simulink model "Proiect"  (R2023b)
settings: Solver=ode45  StartTime=0.0  StopTime=3600  RelTol=1e-3
values from neighbouring files (symbols this model uses):
  A = 332.5    [Proiect.m]
  C = 5.75    [Proiect.m]
  h = 12.99    [Proiect.m]
  h0 = 10.22    [Proiect.m]
  k = 0.025    [Proiect.m]
  k1 = 0.654    [Proiect.m]
  k11 = k2^2 + 4 * (k - k3) * k1    (= 0.0671946)    [Proiect.m]
  k12 = 8 * (k - k3)    (= 0.2048)    [Proiect.m]
  k13 = 2 * (k - k3)    (= 0.0512)    [Proiect.m]
  k2 = -0.015    [Proiect.m]
  k3 = -0.0006    [Proiect.m]
  k_compensare = kpFF/kp_comp    (= 0.13698630137)    [Proiect.m]
  k_eta = 8 * 10^(-5)    (= 8e-05)    [Proiect.m]
  ki2 = 0.184    [Proiect.m]
  kr = 2.1661    [Proiect.m]
  kr1 = Tf1/(kf1*T01)    (= 0.30303030303)    [Proiect.m]
  kr2 = Tf2/(kf2*T02)    (= 47.4368231047)    [Proiect.m]
  kre2 = 47.4    [Proiect.m]
  kri2 = 0.303    [Proiect.m]
  q = 32.45    [Proiect.m]
  q0 = 28.8    [Proiect.m]
  Ti = kr * 1/0.01589    (= 136.31843927)    [Proiect.m]
  Tr1 = Tf1    (= 0.76)    [Proiect.m]
  Tr2 = Tf2    (= 258.25)    [Proiect.m]
  u0 = 4.5    [Proiect.m]
libraries: slpidlib x12
(part 1 of 2)
settings Model: Creator=raluc  LastModifiedBy=raluc
settings ModelReferenceCC: EnableRefExpFcnMdlSchedulingChecks=on

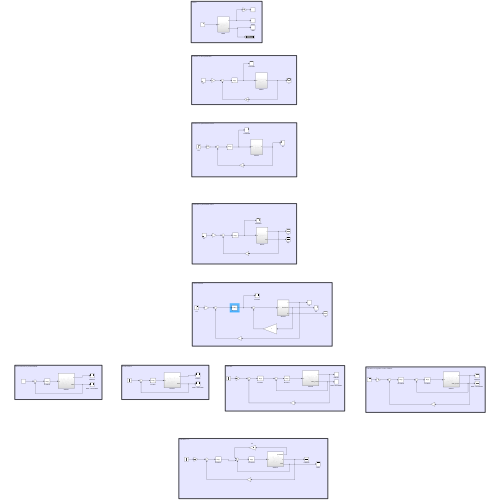
[thumbnail: Simulink's stored preview of the top-level diagram]
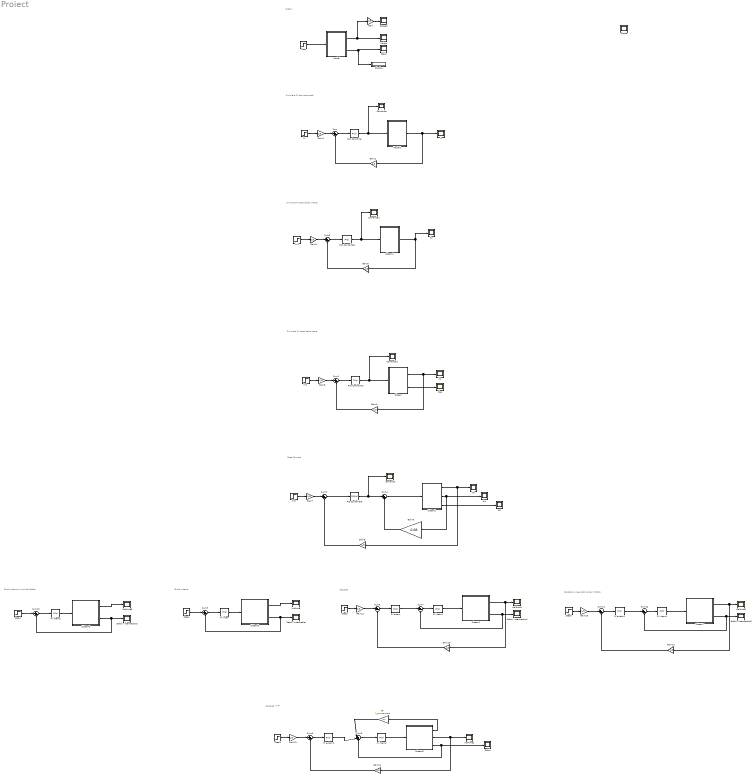
== system Proiect ==
  note: Cascada + FF
  note: Cascada
  note: Bucla Interna
  note: Feed Forward
  note: Simulare PI perturbatie intrare
  note: Simulare PI perturbatie iesire
  note: Simulare PI fara perturbatii
  note: Sistem
  note: Bucla Interna cu pid de Matlab
  note: Cascada cu regulator extern Matlab
  Comanda : Scope
  Comanda1 : Scope
  Comanda2 : Scope
  Debit : Scope
  Debit - intermediar{,1..3} (4 alike) : Scope
  Display : Display
  FF : Gain  Gain=k_compensare
  Gain{,1..8,10..15} (15 alike) : Gain  Gain=1/3
  Gain9 : Gain  Gain=0.08
  Inaltime{,1..4} (5 alike) : Scope
  Model : Subsystem
  Model1 : Subsystem
  PI extern : slpidlib/PID Controller  Controller=PI  Form=Parallel  TimeDomain=Continuous-time  UseExternalTs=off  SampleTime=-1  IntegratorMethod=Forward Euler  FilterMethod=Forward Euler  ControllerParametersSource=internal  P=kr2  I=kr2/Tr2  UseKiTs=off  D=0  N=100  UseFilter=on  TunerSelectOption=Transfer Function Based (PID Tuner App)  InitialConditionSource=internal  InitialConditionForIntegrator=q0  InitialConditionForFilter=0  DifferentiatorICPrevScaledInput=0  ExternalReset=none  TrackingMode=off  Kt=1  LimitOutput=off  SatLimitsSource=internal  UpperSaturationLimit=inf  LowerSaturationLimit=-inf  LinearizeAsGain=on  AntiWindupMode=none  Kb=1  LimitIntegrator=off  UpperIntegratorSaturationLimit=inf  LowerIntegratorSaturationLimit=-inf  POutMin=[]  POutMax=[]  IOutMin=[]  IOutMax=[]  DOutMin=[]  DOutMax=[]  NOutMin=[]  NOutMax=[]  SumOutMin=[]  SumOutMax=[]  SaturationOutMin=[]  SaturationOutMax=[]  PParamMin=[]  PParamMax=[]  IParamMin=[]  IParamMax=[]  DParamMin=[]  DParamMax=[]  NParamMin=[]  NParamMax=[]  KbParamMin=[]  KbParamMax=[]  KtParamMin=[]  KtParamMax=[]  KbOutMin=[]  KbOutMax=[]  KtOutMin=[]  KtOutMax=[]  IntegratorOutMin=[]  IntegratorOutMax=[]  FilterOutMin=[]  FilterOutMax=[]  SumI1OutMin=[]  SumI1OutMax=[]  SumI2OutMin=[]  SumI2OutMax=[]  SumI3OutMin=[]  SumI3OutMax=[]  SumI4OutMin=[]  SumI4OutMax=[]  SumDOutMin=[]  SumDOutMax=[]  DifferentiatorOutMin=[]  DifferentiatorOutMax=[]  FilterDiffOutCoefMin=[]  FilterDiffOutCoefMax=[]  ReciprocalOutMin=[]  ReciprocalOutMax=[]  SumDenOutMin=[]  SumDenOutMax=[]  SumNumOutMin=[]  SumNumOutMax=[]  DivideOutMin=[]  DivideOutMax=[]  UdiffTsProdOutMin=[]  UdiffTsProdOutMax=[]  NTsProdOutMin=[]  NTsProdOutMax=[]  UintegralTsProdOutMin=[]  UintegralTsProdOutMax=[]  UngainTsProdOutMin=[]  UngainTsProdOutMax=[]  ClampingZeroOutDataTypeStr=Inherit: Inherit via back propagation  ClampingZeroOutMin=[]  ClampingZeroOutMax=[]  FilterDenConstantOutDataTypeStr=Inherit: Inherit via back propagation  FilterDenConstantOutMin=[]  FilterDenConstantOutMax=[]  PCopyOutDataTypeStr=Inherit: Inherit via back propagation  PCopyOutMin=[]  PCopyOutMax=[]  NCopyOutDataTypeStr=Inherit: Inherit via back propagation  NCopyOutMin=[]  NCopyOutMax=[]  IntegratorContinuousStateAttributes=''  IntegratorStateMustResolveToSignalObject=off  IntegratorRTWStateStorageClass=Auto  FilterContinuousStateAttributes=''  FilterStateMustResolveToSignalObject=off  FilterRTWStateStorageClass=Auto  ParallelPVariant=InternalParameters  IdealPVariant=Disabled  IVariant=InternalParameters  DVariant=Disabled  IntegratorVariant=Continuous  SatVariant=Disabled  AWVariant=Passthrough  PCopyVariant=Disabled  TRVariant=Disabled  FdbkBlocksVariant=Forward  IdealPFdbkVariant=Disabled  SatFdbkVariant=Disabled  DerivativeFilterVariant=Disabled  NVariant=Disabled  NCopyVariant=Disabled_SignalSpec  FilterICVariant=Disabled  IntegratorICVariant=InternalICs  ExternalResetVariant=Disabled  TRSumVariant=Passthrough  SumFdbkVariant=Disabled  SumVariant=Sum_PI  TsampFilterVariant=InternalTs  TsampNgainVariant=Passthrough  TsampIntegralVariant=Disabled_SignalSpec  ExternalSaturationOutDataTypeStr=Inherit: Same as second input
  PI extern1 : slpidlib/PID Controller  Controller=PI  Form=Parallel  TimeDomain=Continuous-time  UseExternalTs=off  SampleTime=-1  IntegratorMethod=Forward Euler  FilterMethod=Forward Euler  ControllerParametersSource=internal  P=kre2  I=ki2  UseKiTs=off  D=0  N=100  UseFilter=on  TunerSelectOption=Transfer Function Based (PID Tuner App)  InitialConditionSource=internal  InitialConditionForIntegrator=q0  InitialConditionForFilter=0  DifferentiatorICPrevScaledInput=0  ExternalReset=none  TrackingMode=off  Kt=1  LimitOutput=off  SatLimitsSource=internal  UpperSaturationLimit=inf  LowerSaturationLimit=-inf  LinearizeAsGain=on  AntiWindupMode=none  Kb=1  LimitIntegrator=off  UpperIntegratorSaturationLimit=inf  LowerIntegratorSaturationLimit=-inf  POutMin=[]  POutMax=[]  IOutMin=[]  IOutMax=[]  DOutMin=[]  DOutMax=[]  NOutMin=[]  NOutMax=[]  SumOutMin=[]  SumOutMax=[]  SaturationOutMin=[]  SaturationOutMax=[]  PParamMin=[]  PParamMax=[]  IParamMin=[]  IParamMax=[]  DParamMin=[]  DParamMax=[]  NParamMin=[]  NParamMax=[]  KbParamMin=[]  KbParamMax=[]  KtParamMin=[]  KtParamMax=[]  KbOutMin=[]  KbOutMax=[]  KtOutMin=[]  KtOutMax=[]  IntegratorOutMin=[]  IntegratorOutMax=[]  FilterOutMin=[]  FilterOutMax=[]  SumI1OutMin=[]  SumI1OutMax=[]  SumI2OutMin=[]  SumI2OutMax=[]  SumI3OutMin=[]  SumI3OutMax=[]  SumI4OutMin=[]  SumI4OutMax=[]  SumDOutMin=[]  SumDOutMax=[]  DifferentiatorOutMin=[]  DifferentiatorOutMax=[]  FilterDiffOutCoefMin=[]  FilterDiffOutCoefMax=[]  ReciprocalOutMin=[]  ReciprocalOutMax=[]  SumDenOutMin=[]  SumDenOutMax=[]  SumNumOutMin=[]  SumNumOutMax=[]  DivideOutMin=[]  DivideOutMax=[]  UdiffTsProdOutMin=[]  UdiffTsProdOutMax=[]  NTsProdOutMin=[]  NTsProdOutMax=[]  UintegralTsProdOutMin=[]  UintegralTsProdOutMax=[]  UngainTsProdOutMin=[]  UngainTsProdOutMax=[]  ClampingZeroOutDataTypeStr=Inherit: Inherit via back propagation  ClampingZeroOutMin=[]  ClampingZeroOutMax=[]  FilterDenConstantOutDataTypeStr=Inherit: Inherit via back propagation  FilterDenConstantOutMin=[]  FilterDenConstantOutMax=[]  PCopyOutDataTypeStr=Inherit: Inherit via back propagation  PCopyOutMin=[]  PCopyOutMax=[]  NCopyOutDataTypeStr=Inherit: Inherit via back propagation  NCopyOutMin=[]  NCopyOutMax=[]  IntegratorContinuousStateAttributes=''  IntegratorStateMustResolveToSignalObject=off  IntegratorRTWStateStorageClass=Auto  FilterContinuousStateAttributes=''  FilterStateMustResolveToSignalObject=off  FilterRTWStateStorageClass=Auto  ParallelPVariant=InternalParameters  IdealPVariant=Disabled  IVariant=InternalParameters  DVariant=Disabled  IntegratorVariant=Continuous  SatVariant=Disabled  AWVariant=Passthrough  PCopyVariant=Disabled  TRVariant=Disabled  FdbkBlocksVariant=Forward  IdealPFdbkVariant=Disabled  SatFdbkVariant=Disabled  DerivativeFilterVariant=Disabled  NVariant=Disabled  NCopyVariant=Disabled_SignalSpec  FilterICVariant=Disabled  IntegratorICVariant=InternalICs  ExternalResetVariant=Disabled  TRSumVariant=Passthrough  SumFdbkVariant=Disabled  SumVariant=Sum_PI  TsampFilterVariant=InternalTs  TsampNgainVariant=Passthrough  TsampIntegralVariant=Disabled_SignalSpec  ExternalSaturationOutDataTypeStr=Inherit: Same as second input
  PI extern2 : slpidlib/PID Controller  Controller=PI  Form=Parallel  TimeDomain=Continuous-time  UseExternalTs=off  SampleTime=-1  IntegratorMethod=Forward Euler  FilterMethod=Forward Euler  ControllerParametersSource=internal  P=kre2  I=ki2  UseKiTs=off  D=0  N=100  UseFilter=on  TunerSelectOption=Transfer Function Based (PID Tuner App)  InitialConditionSource=internal  InitialConditionForIntegrator=q0  InitialConditionForFilter=0  DifferentiatorICPrevScaledInput=0  ExternalReset=none  TrackingMode=off  Kt=1  LimitOutput=off  SatLimitsSource=internal  UpperSaturationLimit=inf  LowerSaturationLimit=-inf  LinearizeAsGain=on  AntiWindupMode=none  Kb=1  LimitIntegrator=off  UpperIntegratorSaturationLimit=inf  LowerIntegratorSaturationLimit=-inf  POutMin=[]  POutMax=[]  IOutMin=[]  IOutMax=[]  DOutMin=[]  DOutMax=[]  NOutMin=[]  NOutMax=[]  SumOutMin=[]  SumOutMax=[]  SaturationOutMin=[]  SaturationOutMax=[]  PParamMin=[]  PParamMax=[]  IParamMin=[]  IParamMax=[]  DParamMin=[]  DParamMax=[]  NParamMin=[]  NParamMax=[]  KbParamMin=[]  KbParamMax=[]  KtParamMin=[]  KtParamMax=[]  KbOutMin=[]  KbOutMax=[]  KtOutMin=[]  KtOutMax=[]  IntegratorOutMin=[]  IntegratorOutMax=[]  FilterOutMin=[]  FilterOutMax=[]  SumI1OutMin=[]  SumI1OutMax=[]  SumI2OutMin=[]  SumI2OutMax=[]  SumI3OutMin=[]  SumI3OutMax=[]  SumI4OutMin=[]  SumI4OutMax=[]  SumDOutMin=[]  SumDOutMax=[]  DifferentiatorOutMin=[]  DifferentiatorOutMax=[]  FilterDiffOutCoefMin=[]  FilterDiffOutCoefMax=[]  ReciprocalOutMin=[]  ReciprocalOutMax=[]  SumDenOutMin=[]  SumDenOutMax=[]  SumNumOutMin=[]  SumNumOutMax=[]  DivideOutMin=[]  DivideOutMax=[]  UdiffTsProdOutMin=[]  UdiffTsProdOutMax=[]  NTsProdOutMin=[]  NTsProdOutMax=[]  UintegralTsProdOutMin=[]  UintegralTsProdOutMax=[]  UngainTsProdOutMin=[]  UngainTsProdOutMax=[]  ClampingZeroOutDataTypeStr=Inherit: Inherit via back propagation  ClampingZeroOutMin=[]  ClampingZeroOutMax=[]  FilterDenConstantOutDataTypeStr=Inherit: Inherit via back propagation  FilterDenConstantOutMin=[]  FilterDenConstantOutMax=[]  PCopyOutDataTypeStr=Inherit: Inherit via back propagation  PCopyOutMin=[]  PCopyOutMax=[]  NCopyOutDataTypeStr=Inherit: Inherit via back propagation  NCopyOutMin=[]  NCopyOutMax=[]  IntegratorContinuousStateAttributes=''  IntegratorStateMustResolveToSignalObject=off  IntegratorRTWStateStorageClass=Auto  FilterContinuousStateAttributes=''  FilterStateMustResolveToSignalObject=off  FilterRTWStateStorageClass=Auto  ParallelPVariant=InternalParameters  IdealPVariant=Disabled  IVariant=InternalParameters  DVariant=Disabled  IntegratorVariant=Continuous  SatVariant=Disabled  AWVariant=Passthrough  PCopyVariant=Disabled  TRVariant=Disabled  FdbkBlocksVariant=Forward  IdealPFdbkVariant=Disabled  SatFdbkVariant=Disabled  DerivativeFilterVariant=Disabled  NVariant=Disabled  NCopyVariant=Disabled_SignalSpec  FilterICVariant=Disabled  IntegratorICVariant=InternalICs  ExternalResetVariant=Disabled  TRSumVariant=Passthrough  SumFdbkVariant=Disabled  SumVariant=Sum_PI  TsampFilterVariant=InternalTs  TsampNgainVariant=Passthrough  TsampIntegralVariant=Disabled_SignalSpec  ExternalSaturationOutDataTypeStr=Inherit: Same as second input
  PI intern{,1..2,4} (4 alike) : slpidlib/PID Controller  Controller=PI  Form=Parallel  TimeDomain=Continuous-time  UseExternalTs=off  SampleTime=-1  IntegratorMethod=Forward Euler  FilterMethod=Forward Euler  ControllerParametersSource=internal  P=kr1  I=kr1/Tr1  UseKiTs=off  D=0  N=100  UseFilter=on  TunerSelectOption=Transfer Function Based (PID Tuner App)  InitialConditionSource=internal  InitialConditionForIntegrator=4.5  InitialConditionForFilter=0  DifferentiatorICPrevScaledInput=0  ExternalReset=none  TrackingMode=off  Kt=1  LimitOutput=off  SatLimitsSource=internal  UpperSaturationLimit=inf  LowerSaturationLimit=-inf  LinearizeAsGain=on  AntiWindupMode=none  Kb=1  LimitIntegrator=off  UpperIntegratorSaturationLimit=inf  LowerIntegratorSaturationLimit=-inf  POutMin=[]  POutMax=[]  IOutMin=[]  IOutMax=[]  DOutMin=[]  DOutMax=[]  NOutMin=[]  NOutMax=[]  SumOutMin=[]  SumOutMax=[]  SaturationOutMin=[]  SaturationOutMax=[]  PParamMin=[]  PParamMax=[]  IParamMin=[]  IParamMax=[]  DParamMin=[]  DParamMax=[]  NParamMin=[]  NParamMax=[]  KbParamMin=[]  KbParamMax=[]  KtParamMin=[]  KtParamMax=[]  KbOutMin=[]  KbOutMax=[]  KtOutMin=[]  KtOutMax=[]  IntegratorOutMin=[]  IntegratorOutMax=[]  FilterOutMin=[]  FilterOutMax=[]  SumI1OutMin=[]  SumI1OutMax=[]  SumI2OutMin=[]  SumI2OutMax=[]  SumI3OutMin=[]  SumI3OutMax=[]  SumI4OutMin=[]  SumI4OutMax=[]  SumDOutMin=[]  SumDOutMax=[]  DifferentiatorOutMin=[]  DifferentiatorOutMax=[]  FilterDiffOutCoefMin=[]  FilterDiffOutCoefMax=[]  ReciprocalOutMin=[]  ReciprocalOutMax=[]  SumDenOutMin=[]  SumDenOutMax=[]  SumNumOutMin=[]  SumNumOutMax=[]  DivideOutMin=[]  DivideOutMax=[]  UdiffTsProdOutMin=[]  UdiffTsProdOutMax=[]  NTsProdOutMin=[]  NTsProdOutMax=[]  UintegralTsProdOutMin=[]  UintegralTsProdOutMax=[]  UngainTsProdOutMin=[]  UngainTsProdOutMax=[]  ClampingZeroOutDataTypeStr=Inherit: Inherit via back propagation  ClampingZeroOutMin=[]  ClampingZeroOutMax=[]  FilterDenConstantOutDataTypeStr=Inherit: Inherit via back propagation  FilterDenConstantOutMin=[]  FilterDenConstantOutMax=[]  PCopyOutDataTypeStr=Inherit: Inherit via back propagation  PCopyOutMin=[]  PCopyOutMax=[]  NCopyOutDataTypeStr=Inherit: Inherit via back propagation  NCopyOutMin=[]  NCopyOutMax=[]  IntegratorContinuousStateAttributes=''  IntegratorStateMustResolveToSignalObject=off  IntegratorRTWStateStorageClass=Auto  FilterContinuousStateAttributes=''  FilterStateMustResolveToSignalObject=off  FilterRTWStateStorageClass=Auto  ParallelPVariant=InternalParameters  IdealPVariant=Disabled  IVariant=InternalParameters  DVariant=Disabled  IntegratorVariant=Continuous  SatVariant=Disabled  AWVariant=Passthrough  PCopyVariant=Disabled  TRVariant=Disabled  FdbkBlocksVariant=Forward  IdealPFdbkVariant=Disabled  SatFdbkVariant=Disabled  DerivativeFilterVariant=Disabled  NVariant=Disabled  NCopyVariant=Disabled_SignalSpec  FilterICVariant=Disabled  IntegratorICVariant=InternalICs  ExternalResetVariant=Disabled  TRSumVariant=Passthrough  SumFdbkVariant=Disabled  SumVariant=Sum_PI  TsampFilterVariant=InternalTs  TsampNgainVariant=Passthrough  TsampIntegralVariant=Disabled_SignalSpec  ExternalSaturationOutDataTypeStr=Inherit: Same as second input
  PI intern3 : slpidlib/PID Controller  Controller=PI  Form=Parallel  TimeDomain=Continuous-time  UseExternalTs=off  SampleTime=-1  IntegratorMethod=Forward Euler  FilterMethod=Forward Euler  ControllerParametersSource=internal  P=kri2  I=ki2  UseKiTs=off  D=0  N=100  UseFilter=on  TunerSelectOption=Transfer Function Based (PID Tuner App)  InitialConditionSource=internal  InitialConditionForIntegrator=4.5  InitialConditionForFilter=0  DifferentiatorICPrevScaledInput=0  ExternalReset=none  TrackingMode=off  Kt=1  LimitOutput=off  SatLimitsSource=internal  UpperSaturationLimit=inf  LowerSaturationLimit=-inf  LinearizeAsGain=on  AntiWindupMode=none  Kb=1  LimitIntegrator=off  UpperIntegratorSaturationLimit=inf  LowerIntegratorSaturationLimit=-inf  POutMin=[]  POutMax=[]  IOutMin=[]  IOutMax=[]  DOutMin=[]  DOutMax=[]  NOutMin=[]  NOutMax=[]  SumOutMin=[]  SumOutMax=[]  SaturationOutMin=[]  SaturationOutMax=[]  PParamMin=[]  PParamMax=[]  IParamMin=[]  IParamMax=[]  DParamMin=[]  DParamMax=[]  NParamMin=[]  NParamMax=[]  KbParamMin=[]  KbParamMax=[]  KtParamMin=[]  KtParamMax=[]  KbOutMin=[]  KbOutMax=[]  KtOutMin=[]  KtOutMax=[]  IntegratorOutMin=[]  IntegratorOutMax=[]  FilterOutMin=[]  FilterOutMax=[]  SumI1OutMin=[]  SumI1OutMax=[]  SumI2OutMin=[]  SumI2OutMax=[]  SumI3OutMin=[]  SumI3OutMax=[]  SumI4OutMin=[]  SumI4OutMax=[]  SumDOutMin=[]  SumDOutMax=[]  DifferentiatorOutMin=[]  DifferentiatorOutMax=[]  FilterDiffOutCoefMin=[]  FilterDiffOutCoefMax=[]  ReciprocalOutMin=[]  ReciprocalOutMax=[]  SumDenOutMin=[]  SumDenOutMax=[]  SumNumOutMin=[]  SumNumOutMax=[]  DivideOutMin=[]  DivideOutMax=[]  UdiffTsProdOutMin=[]  UdiffTsProdOutMax=[]  NTsProdOutMin=[]  NTsProdOutMax=[]  UintegralTsProdOutMin=[]  UintegralTsProdOutMax=[]  UngainTsProdOutMin=[]  UngainTsProdOutMax=[]  ClampingZeroOutDataTypeStr=Inherit: Inherit via back propagation  ClampingZeroOutMin=[]  ClampingZeroOutMax=[]  FilterDenConstantOutDataTypeStr=Inherit: Inherit via back propagation  FilterDenConstantOutMin=[]  FilterDenConstantOutMax=[]  PCopyOutDataTypeStr=Inherit: Inherit via back propagation  PCopyOutMin=[]  PCopyOutMax=[]  NCopyOutDataTypeStr=Inherit: Inherit via back propagation  NCopyOutMin=[]  NCopyOutMax=[]  IntegratorContinuousStateAttributes=''  IntegratorStateMustResolveToSignalObject=off  IntegratorRTWStateStorageClass=Auto  FilterContinuousStateAttributes=''  FilterStateMustResolveToSignalObject=off  FilterRTWStateStorageClass=Auto  ParallelPVariant=InternalParameters  IdealPVariant=Disabled  IVariant=InternalParameters  DVariant=Disabled  IntegratorVariant=Continuous  SatVariant=Disabled  AWVariant=Passthrough  PCopyVariant=Disabled  TRVariant=Disabled  FdbkBlocksVariant=Forward  IdealPFdbkVariant=Disabled  SatFdbkVariant=Disabled  DerivativeFilterVariant=Disabled  NVariant=Disabled  NCopyVariant=Disabled_SignalSpec  FilterICVariant=Disabled  IntegratorICVariant=InternalICs  ExternalResetVariant=Disabled  TRSumVariant=Passthrough  SumFdbkVariant=Disabled  SumVariant=Sum_PI  TsampFilterVariant=InternalTs  TsampNgainVariant=Passthrough  TsampIntegralVariant=Disabled_SignalSpec  ExternalSaturationOutDataTypeStr=Inherit: Same as second input
  PID Controller : slpidlib/PID Controller  Controller=PI  Form=Parallel  TimeDomain=Continuous-time  UseExternalTs=off  SampleTime=-1  IntegratorMethod=Forward Euler  FilterMethod=Forward Euler  ControllerParametersSource=internal  P=kr  I=kr/Ti  UseKiTs=off  D=0  N=100  UseFilter=on  TunerSelectOption=Transfer Function Based (PID Tuner App)  InitialConditionSource=internal  InitialConditionForIntegrator=u0  InitialConditionForFilter=0  DifferentiatorICPrevScaledInput=0  ExternalReset=none  TrackingMode=off  Kt=1  LimitOutput=off  SatLimitsSource=internal  UpperSaturationLimit=inf  LowerSaturationLimit=-inf  LinearizeAsGain=on  AntiWindupMode=none  Kb=1  LimitIntegrator=off  UpperIntegratorSaturationLimit=inf  LowerIntegratorSaturationLimit=-inf  POutMin=[]  POutMax=[]  IOutMin=[]  IOutMax=[]  DOutMin=[]  DOutMax=[]  NOutMin=[]  NOutMax=[]  SumOutMin=[]  SumOutMax=[]  SaturationOutMin=[]  SaturationOutMax=[]  PParamMin=[]  PParamMax=[]  IParamMin=[]  IParamMax=[]  DParamMin=[]  DParamMax=[]  NParamMin=[]  NParamMax=[]  KbParamMin=[]  KbParamMax=[]  KtParamMin=[]  KtParamMax=[]  KbOutMin=[]  KbOutMax=[]  KtOutMin=[]  KtOutMax=[]  IntegratorOutMin=[]  IntegratorOutMax=[]  FilterOutMin=[]  FilterOutMax=[]  SumI1OutMin=[]  SumI1OutMax=[]  SumI2OutMin=[]  SumI2OutMax=[]  SumI3OutMin=[]  SumI3OutMax=[]  SumI4OutMin=[]  SumI4OutMax=[]  SumDOutMin=[]  SumDOutMax=[]  DifferentiatorOutMin=[]  DifferentiatorOutMax=[]  FilterDiffOutCoefMin=[]  FilterDiffOutCoefMax=[]  ReciprocalOutMin=[]  ReciprocalOutMax=[]  SumDenOutMin=[]  SumDenOutMax=[]  SumNumOutMin=[]  SumNumOutMax=[]  DivideOutMin=[]  DivideOutMax=[]  UdiffTsProdOutMin=[]  UdiffTsProdOutMax=[]  NTsProdOutMin=[]  NTsProdOutMax=[]  UintegralTsProdOutMin=[]  UintegralTsProdOutMax=[]  UngainTsProdOutMin=[]  UngainTsProdOutMax=[]  ClampingZeroOutDataTypeStr=Inherit: Inherit via back propagation  ClampingZeroOutMin=[]  ClampingZeroOutMax=[]  FilterDenConstantOutDataTypeStr=Inherit: Inherit via back propagation  FilterDenConstantOutMin=[]  FilterDenConstantOutMax=[]  PCopyOutDataTypeStr=Inherit: Inherit via back propagation  PCopyOutMin=[]  PCopyOutMax=[]  NCopyOutDataTypeStr=Inherit: Inherit via back propagation  NCopyOutMin=[]  NCopyOutMax=[]  IntegratorContinuousStateAttributes=''  IntegratorStateMustResolveToSignalObject=off  IntegratorRTWStateStorageClass=Auto  FilterContinuousStateAttributes=''  FilterStateMustResolveToSignalObject=off  FilterRTWStateStorageClass=Auto  ParallelPVariant=InternalParameters  IdealPVariant=Disabled  IVariant=InternalParameters  DVariant=Disabled  IntegratorVariant=Continuous  SatVariant=Disabled  AWVariant=Passthrough  PCopyVariant=Disabled  TRVariant=Disabled  FdbkBlocksVariant=Forward  IdealPFdbkVariant=Disabled  SatFdbkVariant=Disabled  DerivativeFilterVariant=Disabled  NVariant=Disabled  NCopyVariant=Disabled_SignalSpec  FilterICVariant=Disabled  IntegratorICVariant=InternalICs  ExternalResetVariant=Disabled  TRSumVariant=Passthrough  SumFdbkVariant=Disabled  SumVariant=Sum_PI  TsampFilterVariant=InternalTs  TsampNgainVariant=Passthrough  TsampIntegralVariant=Disabled_SignalSpec  ExternalSaturationOutDataTypeStr=Inherit: Same as second input
  PID Controller1 : slpidlib/PID Controller  Controller=PI  Form=Parallel  TimeDomain=Continuous-time  UseExternalTs=off  SampleTime=-1  IntegratorMethod=Forward Euler  FilterMethod=Forward Euler  ControllerParametersSource=internal  P=kr  I=kr/Ti  UseKiTs=off  D=0  N=100  UseFilter=on  TunerSelectOption=Transfer Function Based (PID Tuner App)  InitialConditionSource=internal  InitialConditionForIntegrator=4.5  InitialConditionForFilter=0  DifferentiatorICPrevScaledInput=0  ExternalReset=none  TrackingMode=off  Kt=1  LimitOutput=off  SatLimitsSource=internal  UpperSaturationLimit=inf  LowerSaturationLimit=-inf  LinearizeAsGain=on  AntiWindupMode=none  Kb=1  LimitIntegrator=off  UpperIntegratorSaturationLimit=inf  LowerIntegratorSaturationLimit=-inf  POutMin=[]  POutMax=[]  IOutMin=[]  IOutMax=[]  DOutMin=[]  DOutMax=[]  NOutMin=[]  NOutMax=[]  SumOutMin=[]  SumOutMax=[]  SaturationOutMin=[]  SaturationOutMax=[]  PParamMin=[]  PParamMax=[]  IParamMin=[]  IParamMax=[]  DParamMin=[]  DParamMax=[]  NParamMin=[]  NParamMax=[]  KbParamMin=[]  KbParamMax=[]  KtParamMin=[]  KtParamMax=[]  KbOutMin=[]  KbOutMax=[]  KtOutMin=[]  KtOutMax=[]  IntegratorOutMin=[]  IntegratorOutMax=[]  FilterOutMin=[]  FilterOutMax=[]  SumI1OutMin=[]  SumI1OutMax=[]  SumI2OutMin=[]  SumI2OutMax=[]  SumI3OutMin=[]  SumI3OutMax=[]  SumI4OutMin=[]  SumI4OutMax=[]  SumDOutMin=[]  SumDOutMax=[]  DifferentiatorOutMin=[]  DifferentiatorOutMax=[]  FilterDiffOutCoefMin=[]  FilterDiffOutCoefMax=[]  ReciprocalOutMin=[]  ReciprocalOutMax=[]  SumDenOutMin=[]  SumDenOutMax=[]  SumNumOutMin=[]  SumNumOutMax=[]  DivideOutMin=[]  DivideOutMax=[]  UdiffTsProdOutMin=[]  UdiffTsProdOutMax=[]  NTsProdOutMin=[]  NTsProdOutMax=[]  UintegralTsProdOutMin=[]  UintegralTsProdOutMax=[]  UngainTsProdOutMin=[]  UngainTsProdOutMax=[]  ClampingZeroOutDataTypeStr=Inherit: Inherit via back propagation  ClampingZeroOutMin=[]  ClampingZeroOutMax=[]  FilterDenConstantOutDataTypeStr=Inherit: Inherit via back propagation  FilterDenConstantOutMin=[]  FilterDenConstantOutMax=[]  PCopyOutDataTypeStr=Inherit: Inherit via back propagation  PCopyOutMin=[]  PCopyOutMax=[]  NCopyOutDataTypeStr=Inherit: Inherit via back propagation  NCopyOutMin=[]  NCopyOutMax=[]  IntegratorContinuousStateAttributes=''  IntegratorStateMustResolveToSignalObject=off  IntegratorRTWStateStorageClass=Auto  FilterContinuousStateAttributes=''  FilterStateMustResolveToSignalObject=off  FilterRTWStateStorageClass=Auto  ParallelPVariant=InternalParameters  IdealPVariant=Disabled  IVariant=InternalParameters  DVariant=Disabled  IntegratorVariant=Continuous  SatVariant=Disabled  AWVariant=Passthrough  PCopyVariant=Disabled  TRVariant=Disabled  FdbkBlocksVariant=Forward  IdealPFdbkVariant=Disabled  SatFdbkVariant=Disabled  DerivativeFilterVariant=Disabled  NVariant=Disabled  NCopyVariant=Disabled_SignalSpec  FilterICVariant=Disabled  IntegratorICVariant=InternalICs  ExternalResetVariant=Disabled  TRSumVariant=Passthrough  SumFdbkVariant=Disabled  SumVariant=Sum_PI  TsampFilterVariant=InternalTs  TsampNgainVariant=Passthrough  TsampIntegralVariant=Disabled_SignalSpec  ExternalSaturationOutDataTypeStr=Inherit: Same as second input
  PID Controller2 : slpidlib/PID Controller  Controller=PI  Form=Parallel  TimeDomain=Continuous-time  UseExternalTs=off  SampleTime=-1  IntegratorMethod=Forward Euler  FilterMethod=Forward Euler  ControllerParametersSource=internal  P=kr  I=kr/Ti  UseKiTs=off  D=0  N=100  UseFilter=on  TunerSelectOption=Transfer Function Based (PID Tuner App)  InitialConditionSource=internal  InitialConditionForIntegrator=u0  InitialConditionForFilter=0  DifferentiatorICPrevScaledInput=0  ExternalReset=none  TrackingMode=off  Kt=1  LimitOutput=off  SatLimitsSource=internal  UpperSaturationLimit=inf  LowerSaturationLimit=-inf  LinearizeAsGain=on  AntiWindupMode=none  Kb=1  LimitIntegrator=off  UpperIntegratorSaturationLimit=inf  LowerIntegratorSaturationLimit=-inf  POutMin=[]  POutMax=[]  IOutMin=[]  IOutMax=[]  DOutMin=[]  DOutMax=[]  NOutMin=[]  NOutMax=[]  SumOutMin=[]  SumOutMax=[]  SaturationOutMin=[]  SaturationOutMax=[]  PParamMin=[]  PParamMax=[]  IParamMin=[]  IParamMax=[]  DParamMin=[]  DParamMax=[]  NParamMin=[]  NParamMax=[]  KbParamMin=[]  KbParamMax=[]  KtParamMin=[]  KtParamMax=[]  KbOutMin=[]  KbOutMax=[]  KtOutMin=[]  KtOutMax=[]  IntegratorOutMin=[]  IntegratorOutMax=[]  FilterOutMin=[]  FilterOutMax=[]  SumI1OutMin=[]  SumI1OutMax=[]  SumI2OutMin=[]  SumI2OutMax=[]  SumI3OutMin=[]  SumI3OutMax=[]  SumI4OutMin=[]  SumI4OutMax=[]  SumDOutMin=[]  SumDOutMax=[]  DifferentiatorOutMin=[]  DifferentiatorOutMax=[]  FilterDiffOutCoefMin=[]  FilterDiffOutCoefMax=[]  ReciprocalOutMin=[]  ReciprocalOutMax=[]  SumDenOutMin=[]  SumDenOutMax=[]  SumNumOutMin=[]  SumNumOutMax=[]  DivideOutMin=[]  DivideOutMax=[]  UdiffTsProdOutMin=[]  UdiffTsProdOutMax=[]  NTsProdOutMin=[]  NTsProdOutMax=[]  UintegralTsProdOutMin=[]  UintegralTsProdOutMax=[]  UngainTsProdOutMin=[]  UngainTsProdOutMax=[]  ClampingZeroOutDataTypeStr=Inherit: Inherit via back propagation  ClampingZeroOutMin=[]  ClampingZeroOutMax=[]  FilterDenConstantOutDataTypeStr=Inherit: Inherit via back propagation  FilterDenConstantOutMin=[]  FilterDenConstantOutMax=[]  PCopyOutDataTypeStr=Inherit: Inherit via back propagation  PCopyOutMin=[]  PCopyOutMax=[]  NCopyOutDataTypeStr=Inherit: Inherit via back propagation  NCopyOutMin=[]  NCopyOutMax=[]  IntegratorContinuousStateAttributes=''  IntegratorStateMustResolveToSignalObject=off  IntegratorRTWStateStorageClass=Auto  FilterContinuousStateAttributes=''  FilterStateMustResolveToSignalObject=off  FilterRTWStateStorageClass=Auto  ParallelPVariant=InternalParameters  IdealPVariant=Disabled  IVariant=InternalParameters  DVariant=Disabled  IntegratorVariant=Continuous  SatVariant=Disabled  AWVariant=Passthrough  PCopyVariant=Disabled  TRVariant=Disabled  FdbkBlocksVariant=Forward  IdealPFdbkVariant=Disabled  SatFdbkVariant=Disabled  DerivativeFilterVariant=Disabled  NVariant=Disabled  NCopyVariant=Disabled_SignalSpec  FilterICVariant=Disabled  IntegratorICVariant=InternalICs  ExternalResetVariant=Disabled  TRSumVariant=Passthrough  SumFdbkVariant=Disabled  SumVariant=Sum_PI  TsampFilterVariant=InternalTs  TsampNgainVariant=Passthrough  TsampIntegralVariant=Disabled_SignalSpec  ExternalSaturationOutDataTypeStr=Inherit: Same as second input
  PID Controller3 : slpidlib/PID Controller  Controller=PID  Form=Parallel  TimeDomain=Continuous-time  UseExternalTs=off  SampleTime=-1  IntegratorMethod=Forward Euler  FilterMethod=Forward Euler  ControllerParametersSource=internal  P=2.1661  I=0.01589  UseKiTs=off  D=0  N=100  UseFilter=on  TunerSelectOption=Transfer Function Based (PID Tuner App)  InitialConditionSource=internal  InitialConditionForIntegrator=4.5  InitialConditionForFilter=0  DifferentiatorICPrevScaledInput=0  ExternalReset=none  TrackingMode=off  Kt=1  LimitOutput=off  SatLimitsSource=internal  UpperSaturationLimit=inf  LowerSaturationLimit=-inf  LinearizeAsGain=on  AntiWindupMode=none  Kb=1  LimitIntegrator=off  UpperIntegratorSaturationLimit=inf  LowerIntegratorSaturationLimit=-inf  POutMin=[]  POutMax=[]  IOutMin=[]  IOutMax=[]  DOutMin=[]  DOutMax=[]  NOutMin=[]  NOutMax=[]  SumOutMin=[]  SumOutMax=[]  SaturationOutMin=[]  SaturationOutMax=[]  PParamMin=[]  PParamMax=[]  IParamMin=[]  IParamMax=[]  DParamMin=[]  DParamMax=[]  NParamMin=[]  NParamMax=[]  KbParamMin=[]  KbParamMax=[]  KtParamMin=[]  KtParamMax=[]  KbOutMin=[]  KbOutMax=[]  KtOutMin=[]  KtOutMax=[]  IntegratorOutMin=[]  IntegratorOutMax=[]  FilterOutMin=[]  FilterOutMax=[]  SumI1OutMin=[]  SumI1OutMax=[]  SumI2OutMin=[]  SumI2OutMax=[]  SumI3OutMin=[]  SumI3OutMax=[]  SumI4OutMin=[]  SumI4OutMax=[]  SumDOutMin=[]  SumDOutMax=[]  DifferentiatorOutMin=[]  DifferentiatorOutMax=[]  FilterDiffOutCoefMin=[]  FilterDiffOutCoefMax=[]  ReciprocalOutMin=[]  ReciprocalOutMax=[]  SumDenOutMin=[]  SumDenOutMax=[]  SumNumOutMin=[]  SumNumOutMax=[]  DivideOutMin=[]  DivideOutMax=[]  UdiffTsProdOutMin=[]  UdiffTsProdOutMax=[]  NTsProdOutMin=[]  NTsProdOutMax=[]  UintegralTsProdOutMin=[]  UintegralTsProdOutMax=[]  UngainTsProdOutMin=[]  UngainTsProdOutMax=[]  ClampingZeroOutDataTypeStr=Inherit: Inherit via back propagation  ClampingZeroOutMin=[]  ClampingZeroOutMax=[]  FilterDenConstantOutDataTypeStr=Inherit: Inherit via back propagation  FilterDenConstantOutMin=[]  FilterDenConstantOutMax=[]  PCopyOutDataTypeStr=Inherit: Inherit via back propagation  PCopyOutMin=[]  PCopyOutMax=[]  NCopyOutDataTypeStr=Inherit: Inherit via back propagation  NCopyOutMin=[]  NCopyOutMax=[]  IntegratorContinuousStateAttributes=''  IntegratorStateMustResolveToSignalObject=off  IntegratorRTWStateStorageClass=Auto  FilterContinuousStateAttributes=''  FilterStateMustResolveToSignalObject=off  FilterRTWStateStorageClass=Auto  ParallelPVariant=InternalParameters  IdealPVariant=Disabled  IVariant=InternalParameters  DVariant=InternalParameters  IntegratorVariant=Continuous  SatVariant=Disabled  AWVariant=Passthrough  PCopyVariant=Disabled  TRVariant=Disabled  FdbkBlocksVariant=Forward  IdealPFdbkVariant=Disabled  SatFdbkVariant=Disabled  DerivativeFilterVariant=ContFilter  NVariant=InternalParameters  NCopyVariant=Disabled  FilterICVariant=InternalICsFilter  IntegratorICVariant=InternalICs  ExternalResetVariant=Disabled  TRSumVariant=Passthrough  SumFdbkVariant=Disabled  SumVariant=Sum_PID  TsampFilterVariant=InternalTs  TsampNgainVariant=Passthrough  TsampIntegralVariant=Disabled_SignalSpec  ExternalSaturationOutDataTypeStr=Inherit: Same as second input
  Scope2 : Scope
  Sistem : Subsystem
  Sistem1 : Subsystem
  Sistem2 : Subsystem
  Sistem3 : Subsystem
  Sistem4 : Subsystem
  Sistem5 : Subsystem
  Sistem6 : Subsystem
  Sistem7 : Subsystem
  Step : Step  Time=0  Before=u0  After=u0+0.5  SampleTime=0
  Step1 : Step  Time=0  Before=q0  After=q  SampleTime=0
  Step2 : Step  Time=0  Before=h0  After=h  SampleTime=0
  Step3 : Step  Time=0  Before=h0  After=h  SampleTime=0
  Step4 : Step  Time=0  Before=q0  After=q  SampleTime=0
  Step5 : Step  Time=0  Before=h0  After=h  SampleTime=0
  Sum{,1..3,5..8,10..12} (11 alike) : Sum  Inputs=|+-
  Sum4 : Sum  Inputs=|++
  Sum9 : Sum  Inputs=|++-
  comanda : Scope
  debit : Scope
  dis : Scope
  dqe : Scope
  h{,1..3} (4 alike) : Scope
  h*{,1..3} (4 alike) : Step  Time=0  Before=h0  After=h  SampleTime=0
  height : Scope
  qe : Scope
  Scope : Scope
  wires:
  Step/1 -> Model/1(uc)
  Model/1(h) -> Gain/1, height/1
  Model/2(q) -> debit/1, Display/1
  Gain/1 -> Scope2/1
  h*/1 -> Gain1/1
  PID Controller/1 -> Comanda/1, Model1/1(uc)
  Gain1/1 -> Sum/1
  Model1/1(h) -> h/1, Gain2/1
  Sum/1 -> PID Controller/1
  Gain2/1 -> Sum/2
  Sistem/2(dqe) -> dqe/1
  PID Controller1/1 -> Sistem/1(uc), Comanda1/1
  Sistem/1(h) -> Gain4/1, h1/1
  Sum1/1 -> PID Controller1/1
  Gain4/1 -> Sum1/2
  Gain3/1 -> Sum1/1
  h*1/1 -> Gain3/1
  h*2/1 -> Gain5/1
  Gain6/1 -> Sum2/2
  Sistem1/1(h) -> h2/1, Gain6/1
  PID Controller2/1 -> Comanda2/1, Sistem1/1(uc)
  Sum2/1 -> PID Controller2/1
  Gain5/1 -> Sum2/1
  Sistem2/3(qe) -> qe/1
  Sistem2/1(h) -> Gain8/1, h3/1
  h*3/1 -> Gain7/1
  Gain8/1 -> Sum3/2
  Gain9/1 -> Sum4/2
  PID Controller3/1 -> comanda/1, Sum4/1
  Sum4/1 -> Sistem2/1(uc)
  Gain7/1 -> Sum3/1
  Sum3/1 -> PID Controller3/1
  Sistem2/2(disturbance) -> Gain9/1, dis/1
  Step1/1 -> Sum5/1
  Sum5/1 -> PI intern/1
  Sistem3/1(h) -> Inaltime/1
  PI intern/1 -> Sistem3/1(uc)
  Sistem3/2(debit) -> Debit - intermediar/1, Sum5/2
  PI extern/1 -> Sum7/1
  Gain10/1 -> Sum6/2
  Gain11/1 -> Sum6/1
  PI intern1/1 -> Sistem4/1(uc)
  Step2/1 -> Gain11/1
  Sum6/1 -> PI extern/1
  Sum7/1 -> PI intern1/1
  Sistem4/2(debit_pompa) -> Sum7/2, Debit - intermediar1/1
  Sistem4/1(h) -> Inaltime1/1, Gain10/1
  PI extern1/1 -> Sum9/2
  Sistem5/1(perturbatie) -> FF/1
  FF/1 -> Sum9/1
  Gain13/1 -> Sum8/1
  Sum8/1 -> PI extern1/1
  Sum9/1 -> PI intern2/1
  PI intern2/1 -> Sistem5/1(uc)
  Sistem5/2(h) -> Inaltime2/1, Gain12/1
  Sistem5/3(debit) -> Debit/1, Sum9/3
  Gain12/1 -> Sum8/2
  Step3/1 -> Gain13/1
  Step4/1 -> Sum10/1
  Sistem6/1(h) -> Inaltime3/1
  Sistem6/2(debit) -> Debit - intermediar2/1, Sum10/2
  PI intern3/1 -> Sistem6/1(uc)
  Sum10/1 -> PI intern3/1
  Gain14/1 -> Sum11/2
  Sistem7/2(debit_pompa) -> Sum12/2, Debit - intermediar3/1
  Sum11/1 -> PI extern2/1
  Sum12/1 -> PI intern4/1
  PI intern4/1 -> Sistem7/1(uc)
  Step5/1 -> Gain15/1
  Gain15/1 -> Sum11/1
  Sistem7/1(h) -> Inaltime4/1, Gain14/1
  PI extern2/1 -> Sum12/1

== system Proiect/Model ==
  uc : Inport
  Amplificator : Subsystem
  Curent Rotoric : Subsystem
  Filtru : Subsystem
  Motor : Subsystem
  Pompa : Subsystem
  Randament Pompa : Subsystem
  Rezervor : Subsystem
  h : Outport
  q : Outport  Port=2
  wires:
  Curent Rotoric/1(im) -> Motor/2(im)
  Motor/1(kn) -> Pompa/1(kn)
  Amplificator/1(um) -> Randament Pompa/2(um), Curent Rotoric/4(um), Motor/1(um)
  uc/1 -> Amplificator/1(ua)
  Randament Pompa/1(eta) -> Curent Rotoric/3(eta)
  Pompa/1(qi) -> Filtru/1(q)
  Filtru/1(q_f) -> Rezervor/1(q), q/1, Randament Pompa/1(q), Curent Rotoric/2(q)
  Rezervor/1(h) -> Pompa/2(h), Curent Rotoric/1(h), h/1

== system Proiect/Model1 ==
  uc : Inport
  Amplificator : Subsystem
  Curent Rotoric : Subsystem
  Filtru : Subsystem
  Motor : Subsystem
  Pompa : Subsystem
  Randament Pompa : Subsystem
  Rezervor : Subsystem
  h : Outport
  wires:
  Curent Rotoric/1(im) -> Motor/2(im)
  Rezervor/1(h) -> h/1, Pompa/2(h), Curent Rotoric/1(h)
  Motor/1(kn) -> Pompa/1(kn)
  Amplificator/1(um) -> Randament Pompa/2(um), Curent Rotoric/4(um), Motor/1(um)
  uc/1 -> Amplificator/1(ua)
  Randament Pompa/1(eta) -> Curent Rotoric/3(eta)
  Pompa/1(qi) -> Filtru/1(q)
  Filtru/1(q_f) -> Randament Pompa/1(q), Curent Rotoric/2(q), Rezervor/1(q)

== system Proiect/Sistem ==
  uc : Inport
  Amplificator : Subsystem
  Curent Rotoric : Subsystem
  Filtru : Subsystem
  Motor : Subsystem
  Pompa : Subsystem
  Randament Pompa : Subsystem
  Rezervor : Subsystem
  h : Outport
  dqe : Outport  Port=2
  wires:
  Curent Rotoric/1(im) -> Motor/2(im)
  Rezervor/1(h) -> Pompa/2(h), Curent Rotoric/1(h), h/1
  Motor/1(kn) -> Pompa/1(kn)
  Amplificator/1(um) -> Randament Pompa/2(um), Curent Rotoric/4(um), Motor/1(um)
  uc/1 -> Amplificator/1(ua)
  Randament Pompa/1(eta) -> Curent Rotoric/3(eta)
  Pompa/1(qi) -> Filtru/1(q)
  Filtru/1(q_f) -> Randament Pompa/1(q), Curent Rotoric/2(q), Rezervor/1(q)
  Rezervor/2(qe) -> dqe/1

== system Proiect/Sistem1 ==
  uc : Inport
  Amplificator : Subsystem
  Curent Rotoric : Subsystem
  Filtru : Subsystem
  Motor : Subsystem
  Pompa : Subsystem
  Randament Pompa : Subsystem
  Rezervor : Subsystem
  perturbation : Step  Time=250  After=0.05  SampleTime=0
  h : Outport
  wires:
  Curent Rotoric/1(im) -> Motor/2(im)
  Rezervor/1(h) -> h/1, Pompa/3(h), Curent Rotoric/1(h)
  Amplificator/1(um) -> Randament Pompa/2(um), Curent Rotoric/4(um), Motor/1(um)
  uc/1 -> Amplificator/1(ua)
  Randament Pompa/1(eta) -> Curent Rotoric/3(eta)
  Filtru/1(q_f) -> Randament Pompa/1(q), Curent Rotoric/2(q), Rezervor/1(q)
  Motor/1(kn) -> Pompa/1(kn)
  Pompa/1(q) -> Filtru/1(q)
  perturbation/1 -> Pompa/2(perturbatie k)

== system Proiect/Sistem2 ==
  uc : Inport
  Amplificator : Subsystem
  Curent Rotoric : Subsystem
  Filtru : Subsystem
  Motor : Subsystem
  Pompa : Subsystem
  Randament Pompa : Subsystem
  Rezervor : Subsystem
  h : Outport
  disturbance : Outport  Port=2
  qe : Outport  Port=3
  wires:
  Curent Rotoric/1(im) -> Motor/2(im)
  Rezervor/1(h) -> Pompa/2(h), Curent Rotoric/1(h), h/1
  Motor/1(kn) -> Pompa/1(kn)
  Amplificator/1(um) -> Randament Pompa/2(um), Curent Rotoric/4(um), Motor/1(um)
  uc/1 -> Amplificator/1(ua)
  Randament Pompa/1(eta) -> Curent Rotoric/3(eta)
  Pompa/1(qi) -> Filtru/1(q)
  Filtru/1(q_f) -> Randament Pompa/1(q), Curent Rotoric/2(q), Rezervor/1(q)
  Rezervor/2(perturbatie) -> disturbance/1
  Rezervor/3(qe) -> qe/1

== system Proiect/Sistem3 ==
  uc : Inport
  Amplificator : Subsystem
  Constant : Constant  Value=0
  Curent Rotoric : Subsystem
  Debit iesire pompa : Scope
  Filtru : Subsystem
  Motor : Subsystem
  Pompa : Subsystem
  Randament Pompa : Subsystem
  Rezervor : Subsystem
  inaltime : Scope
  h : Outport
  debit : Outport  Port=2
  wires:
  Pompa/1(q) -> Filtru/1(q)
  Amplificator/1(um) -> Motor/1(um), Randament Pompa/2(um), Curent Rotoric/4(um)
  Motor/1(kn) -> Pompa/1(kn)
  Randament Pompa/1(eta) -> Curent Rotoric/3(eta)
  Curent Rotoric/1(im) -> Motor/2(im)
  Filtru/1(q_f) -> Debit iesire pompa/1, debit/1, Rezervor/1(q), Randament Pompa/1(q), Curent Rotoric/2(q)
  Constant/1 -> Pompa/2(perturbatie k)
  uc/1 -> Amplificator/1(ua)
  Rezervor/1(h) -> h/1, inaltime/1

== system Proiect/Sistem4 ==
  uc : Inport
  Amplificator : Subsystem
  Constant : Constant  Value=0
  Curent Rotoric : Subsystem
  Filtru : Subsystem
  Motor : Subsystem
  Pompa : Subsystem
  Randament Pompa : Subsystem
  Rezervor : Subsystem
  h : Outport
  debit_pompa : Outport  Port=2
  wires:
  Pompa/1(q) -> Filtru/1(q)
  Amplificator/1(um) -> Motor/1(um), Randament Pompa/2(um), Curent Rotoric/4(um)
  Motor/1(kn) -> Pompa/1(kn)
  Randament Pompa/1(eta) -> Curent Rotoric/3(eta)
  Curent Rotoric/1(im) -> Motor/2(im)
  Filtru/1(q_f) -> debit_pompa/1, Rezervor/1(q), Randament Pompa/1(q), Curent Rotoric/2(q)
  Constant/1 -> Pompa/2(perturbatie k)
  uc/1 -> Amplificator/1(ua)
  Rezervor/1(h) -> Curent Rotoric/1(h), Pompa/3(h), h/1

== system Proiect/Sistem5 ==
  uc : Inport
  Amplificator : Subsystem
  Curent Rotoric : Subsystem
  Debit iesire pompa : Scope
  Filtru : Subsystem
  Motor : Subsystem
  Pompa : Subsystem
  Randament Pompa : Subsystem
  Rezervor : Subsystem
  perturbation : Step  Time=300  After=0.05  SampleTime=0
  perturbatie : Outport
  h : Outport  Port=2
  debit : Outport  Port=3
  wires:
  Pompa/1(q) -> Filtru/1(q)
  Amplificator/1(um) -> Motor/1(um), Randament Pompa/2(um), Curent Rotoric/4(um)
  Motor/1(kn) -> Pompa/1(kn)
  Randament Pompa/1(eta) -> Curent Rotoric/3(eta)
  Curent Rotoric/1(im) -> Motor/2(im)
  Filtru/1(q_f) -> Debit iesire pompa/1, debit/1, Rezervor/1(q), Randament Pompa/1(q), Curent Rotoric/2(q)
  perturbation/1 -> Pompa/2(perturbatie k)
  uc/1 -> Amplificator/1(ua)
  Rezervor/1(h) -> Curent Rotoric/1(h), Pompa/3(h), h/1
  Rezervor/2(perturbatie) -> perturbatie/1

== system Proiect/Sistem6 ==
  uc : Inport
  Amplificator : Subsystem
  Constant : Constant  Value=0
  Curent Rotoric : Subsystem
  Debit iesire pompa : Scope
  Filtru : Subsystem
  Motor : Subsystem
  Pompa : Subsystem
  Randament Pompa : Subsystem
  Rezervor : Subsystem
  inaltime : Scope
  h : Outport
  debit : Outport  Port=2
  wires:
  Pompa/1(q) -> Filtru/1(q)
  Amplificator/1(um) -> Motor/1(um), Randament Pompa/2(um), Curent Rotoric/4(um)
  Motor/1(kn) -> Pompa/1(kn)
  Randament Pompa/1(eta) -> Curent Rotoric/3(eta)
  Curent Rotoric/1(im) -> Motor/2(im)
  Filtru/1(q_f) -> Debit iesire pompa/1, debit/1, Rezervor/1(q), Randament Pompa/1(q), Curent Rotoric/2(q)
  Constant/1 -> Pompa/2(perturbatie k)
  uc/1 -> Amplificator/1(ua)
  Rezervor/1(h) -> h/1, inaltime/1

== system Proiect/Sistem7 ==
  uc : Inport
  Amplificator : Subsystem
  Constant : Constant  Value=0
  Curent Rotoric : Subsystem
  Filtru : Subsystem
  Motor : Subsystem
  Pompa : Subsystem
  Randament Pompa : Subsystem
  Rezervor : Subsystem
  h : Outport
  debit_pompa : Outport  Port=2
  wires:
  Pompa/1(q) -> Filtru/1(q)
  Amplificator/1(um) -> Motor/1(um), Randament Pompa/2(um), Curent Rotoric/4(um)
  Motor/1(kn) -> Pompa/1(kn)
  Randament Pompa/1(eta) -> Curent Rotoric/3(eta)
  Curent Rotoric/1(im) -> Motor/2(im)
  Filtru/1(q_f) -> debit_pompa/1, Rezervor/1(q), Randament Pompa/1(q), Curent Rotoric/2(q)
  Constant/1 -> Pompa/2(perturbatie k)
  uc/1 -> Amplificator/1(ua)
  Rezervor/1(h) -> Curent Rotoric/1(h), Pompa/3(h), h/1

== system Proiect/Model/Amplificator ==
  ua : Inport
  Constant : Constant  Value=8.1
  Gain : Gain  Gain=2.2
  Gain1 : Gain  Gain=2.2
  Gain2 : Gain  Gain=5
  Saturation : Saturate  UpperLimit=22  LowerLimit=0
  Sum : Sum  Inputs=|++
  Sum1 : Sum  Inputs=|+-
  Switch : Switch  Threshold=8.1  SaturateOnIntegerOverflow=off  InputSameDT=off
  um : Outport
  wires:
  Switch/1 -> Saturation/1
  ua/1 -> Switch/2, Gain/1, Sum1/1, Gain1/1
  Gain1/1 -> Sum/1
  Gain2/1 -> Sum/2
  Saturation/1 -> um/1
  Gain/1 -> Switch/3
  Constant/1 -> Sum1/2
  Sum1/1 -> Gain2/1
  Sum/1 -> Switch/1

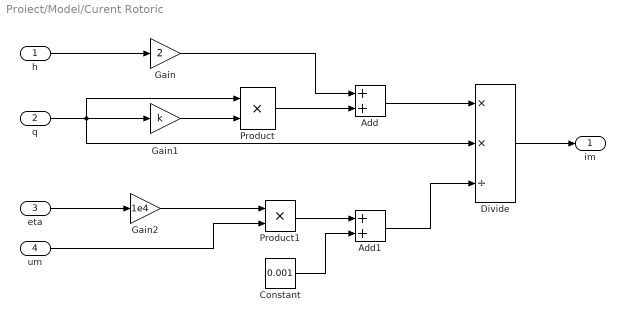
== system Proiect/Model/Curent Rotoric ==
  h : Inport
  q : Inport  Port=2
  eta : Inport  Port=3
  um : Inport  Port=4
  Add : Sum
  Add1 : Sum
  Constant : Constant  Value=0.001
  Divide : Product  Inputs=**/
  Gain : Gain  Gain=2
  Gain1 : Gain  Gain=k
  Gain2 : Gain  Gain=1e4
  Product : Product
  Product1 : Product
  im : Outport
  wires:
  Gain1/1 -> Product/2
  Product/1 -> Add/2
  Gain2/1 -> Product1/1
  h/1 -> Gain/1
  Constant/1 -> Add1/2
  Gain/1 -> Add/1
  um/1 -> Product1/2
  Add1/1 -> Divide/3
  Divide/1 -> im/1
  Add/1 -> Divide/1
  q/1 -> Divide/2, Product/1, Gain1/1
  eta/1 -> Gain2/1
  Product1/1 -> Add1/1

== system Proiect/Model/Filtru ==
  q : Inport
  Integrator : Integrator  InitialCondition=q0
  Sum : Sum  Inputs=|+-
  q_f : Outport
  wires:
  q/1 -> Sum/1
  Integrator/1 -> q_f/1, Sum/2
  Sum/1 -> Integrator/1

== system Proiect/Model/Motor ==
  um : Inport
  im : Inport  Port=2
  Add : Sum  Inputs=+-
  Gain : Gain  Gain=3
  kn : Outport
  wires:
  im/1 -> Gain/1
  um/1 -> Add/1
  Add/1 -> kn/1
  Gain/1 -> Add/2

== system Proiect/Model/Pompa ==
  kn : Inport
  h : Inport  Port=2
  Add : Sum
  Gain : Gain  Gain=k11
  Gain1 : Gain  Gain=k2
  Gain2 : Gain  Gain=1/k13
  Gain3 : Gain  Gain=k12
  Product : Product
  Square Root : Sqrt
  Subtract : Sum  Inputs=+-
  qi : Outport
  wires:
  Gain/1 -> Subtract/1
  Square Root/1 -> Add/2
  Gain3/1 -> Subtract/2
  Product/1 -> Gain/1
  Subtract/1 -> Square Root/1
  Gain2/1 -> qi/1
  kn/1 -> Product/1, Gain1/1, Product/2
  Add/1 -> Gain2/1
  Gain1/1 -> Add/1
  h/1 -> Gain3/1

== system Proiect/Model/Randament Pompa ==
  q : Inport
  um : Inport  Port=2
  Gain : Gain  Gain=k_eta
  Product : Product
  eta : Outport
  wires:
  um/1 -> Gain/1
  Gain/1 -> Product/2
  Product/1 -> eta/1
  q/1 -> Product/1

== system Proiect/Model/Rezervor ==
  q : Inport
  Gain : Gain  Gain=1/A
  Integrator : Integrator  InitialCondition=h0
  Interpreted MATLAB Function : MATLABFcn  MATLABFcn=sqrt(u)*9
  Sum : Sum  Inputs=|+-
  h : Outport
  wires:
  Interpreted MATLAB Function/1 -> Sum/2
  Sum/1 -> Gain/1
  q/1 -> Sum/1
  Gain/1 -> Integrator/1
  Integrator/1 -> Interpreted MATLAB Function/1, h/1

== system Proiect/Model1/Amplificator ==
  ua : Inport
  Constant : Constant  Value=8.1
  Gain : Gain  Gain=2.2
  Gain1 : Gain  Gain=2.2
  Gain2 : Gain  Gain=5
  Saturation : Saturate  UpperLimit=22  LowerLimit=0
  Sum : Sum  Inputs=|++
  Sum1 : Sum  Inputs=|+-
  Switch : Switch  Threshold=8.1  SaturateOnIntegerOverflow=off  InputSameDT=off
  um : Outport
  wires:
  Switch/1 -> Saturation/1
  ua/1 -> Switch/2, Gain/1, Sum1/1, Gain1/1
  Gain1/1 -> Sum/1
  Gain2/1 -> Sum/2
  Saturation/1 -> um/1
  Gain/1 -> Switch/3
  Constant/1 -> Sum1/2
  Sum1/1 -> Gain2/1
  Sum/1 -> Switch/1

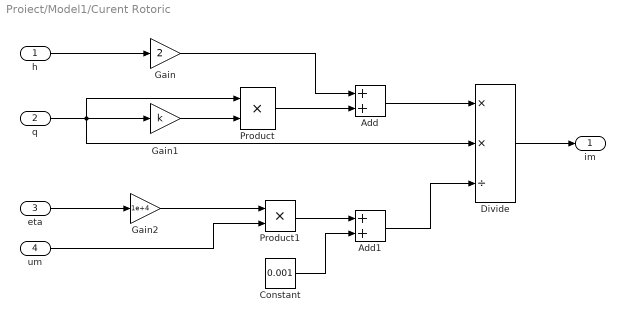
== system Proiect/Model1/Curent Rotoric ==
  h : Inport
  q : Inport  Port=2
  eta : Inport  Port=3
  um : Inport  Port=4
  Add : Sum
  Add1 : Sum
  Constant : Constant  Value=0.001
  Divide : Product  Inputs=**/
  Gain : Gain  Gain=2
  Gain1 : Gain  Gain=k
  Gain2 : Gain  Gain=1e+4
  Product : Product
  Product1 : Product
  im : Outport
  wires:
  Gain1/1 -> Product/2
  Product/1 -> Add/2
  Gain2/1 -> Product1/1
  h/1 -> Gain/1
  Constant/1 -> Add1/2
  Gain/1 -> Add/1
  um/1 -> Product1/2
  Add1/1 -> Divide/3
  Divide/1 -> im/1
  Add/1 -> Divide/1
  q/1 -> Divide/2, Product/1, Gain1/1
  eta/1 -> Gain2/1
  Product1/1 -> Add1/1

== system Proiect/Model1/Filtru ==
  q : Inport
  Integrator : Integrator  InitialCondition=q0
  Sum : Sum  Inputs=|+-
  q_f : Outport
  wires:
  q/1 -> Sum/1
  Integrator/1 -> q_f/1, Sum/2
  Sum/1 -> Integrator/1

== system Proiect/Model1/Motor ==
  um : Inport
  im : Inport  Port=2
  Add : Sum  Inputs=+-
  Gain : Gain  Gain=3
  kn : Outport
  wires:
  im/1 -> Gain/1
  um/1 -> Add/1
  Add/1 -> kn/1
  Gain/1 -> Add/2

== system Proiect/Model1/Pompa ==
  kn : Inport
  h : Inport  Port=2
  Add : Sum
  Gain : Gain  Gain=k11
  Gain1 : Gain  Gain=k2
  Gain2 : Gain  Gain=1/k13
  Gain3 : Gain  Gain=k12
  Product : Product
  Square Root : Sqrt
  Subtract : Sum  Inputs=+-
  qi : Outport
  wires:
  Gain/1 -> Subtract/1
  Square Root/1 -> Add/2
  Gain3/1 -> Subtract/2
  Product/1 -> Gain/1
  Subtract/1 -> Square Root/1
  Gain2/1 -> qi/1
  kn/1 -> Product/1, Gain1/1, Product/2
  Add/1 -> Gain2/1
  Gain1/1 -> Add/1
  h/1 -> Gain3/1

== system Proiect/Model1/Randament Pompa ==
  q : Inport
  um : Inport  Port=2
  Gain : Gain  Gain=k_eta
  Product : Product
  eta : Outport
  wires:
  um/1 -> Gain/1
  Gain/1 -> Product/2
  Product/1 -> eta/1
  q/1 -> Product/1

== system Proiect/Model1/Rezervor ==
  q : Inport
  Gain : Gain  Gain=1/A
  Integrator : Integrator  InitialCondition=h0
  Interpreted MATLAB Function : MATLABFcn  MATLABFcn=sqrt(u)*9
  Sum : Sum  Inputs=|+-
  h : Outport
  wires:
  Sum/1 -> Gain/1
  Integrator/1 -> Interpreted MATLAB Function/1, h/1
  q/1 -> Sum/1
  Gain/1 -> Integrator/1
  Interpreted MATLAB Function/1 -> Sum/2

== system Proiect/Sistem/Amplificator ==
  ua : Inport
  Constant : Constant  Value=8.1
  Gain : Gain  Gain=2.2
  Gain1 : Gain  Gain=2.2
  Gain2 : Gain  Gain=5
  Saturation : Saturate  UpperLimit=22  LowerLimit=0
  Sum : Sum  Inputs=|++
  Sum1 : Sum  Inputs=|+-
  Switch : Switch  Threshold=8.1  SaturateOnIntegerOverflow=off  InputSameDT=off
  um : Outport
  wires:
  Switch/1 -> Saturation/1
  ua/1 -> Switch/2, Gain/1, Sum1/1, Gain1/1
  Gain1/1 -> Sum/1
  Gain2/1 -> Sum/2
  Saturation/1 -> um/1
  Gain/1 -> Switch/3
  Constant/1 -> Sum1/2
  Sum1/1 -> Gain2/1
  Sum/1 -> Switch/1

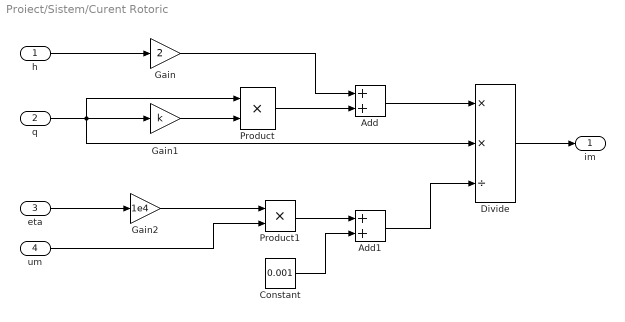
== system Proiect/Sistem/Curent Rotoric ==
  h : Inport
  q : Inport  Port=2
  eta : Inport  Port=3
  um : Inport  Port=4
  Add : Sum
  Add1 : Sum
  Constant : Constant  Value=0.001
  Divide : Product  Inputs=**/
  Gain : Gain  Gain=2
  Gain1 : Gain  Gain=k
  Gain2 : Gain  Gain=1e4
  Product : Product
  Product1 : Product
  im : Outport
  wires:
  Gain1/1 -> Product/2
  Product/1 -> Add/2
  Gain2/1 -> Product1/1
  h/1 -> Gain/1
  Constant/1 -> Add1/2
  Gain/1 -> Add/1
  um/1 -> Product1/2
  Add1/1 -> Divide/3
  Divide/1 -> im/1
  Add/1 -> Divide/1
  q/1 -> Divide/2, Product/1, Gain1/1
  eta/1 -> Gain2/1
  Product1/1 -> Add1/1

== system Proiect/Sistem/Filtru ==
  q : Inport
  Integrator : Integrator  InitialCondition=q0
  Sum : Sum  Inputs=|+-
  q_f : Outport
  wires:
  q/1 -> Sum/1
  Integrator/1 -> q_f/1, Sum/2
  Sum/1 -> Integrator/1

== system Proiect/Sistem/Motor ==
  um : Inport
  im : Inport  Port=2
  Add : Sum  Inputs=+-
  Gain : Gain  Gain=3
  kn : Outport
  wires:
  im/1 -> Gain/1
  um/1 -> Add/1
  Add/1 -> kn/1
  Gain/1 -> Add/2

== system Proiect/Sistem/Pompa ==
  kn : Inport
  h : Inport  Port=2
  Add : Sum
  Gain : Gain  Gain=k11
  Gain1 : Gain  Gain=k2
  Gain2 : Gain  Gain=1/k13
  Gain3 : Gain  Gain=k12
  Product : Product
  Square Root : Sqrt
  Subtract : Sum  Inputs=+-
  qi : Outport
  wires:
  Gain/1 -> Subtract/1
  Square Root/1 -> Add/2
  Gain3/1 -> Subtract/2
  Product/1 -> Gain/1
  Subtract/1 -> Square Root/1
  Gain2/1 -> qi/1
  kn/1 -> Product/1, Gain1/1, Product/2
  Add/1 -> Gain2/1
  Gain1/1 -> Add/1
  h/1 -> Gain3/1

== system Proiect/Sistem/Randament Pompa ==
  q : Inport
  um : Inport  Port=2
  Gain : Gain  Gain=k_eta
  Product : Product
  eta : Outport
  wires:
  um/1 -> Gain/1
  Gain/1 -> Product/2
  Product/1 -> eta/1
  q/1 -> Product/1

== system Proiect/Sistem/Rezervor ==
  q : Inport
  C : Step  Time=250  Before=C  After=8  SampleTime=0
  Gain : Gain  Gain=1/A
  Integrator : Integrator  InitialCondition=h0
  Product : Product
  Square Root : Sqrt
  Sum : Sum  Inputs=|+-
  h : Outport
  qe : Outport  Port=2
  wires:
  Sum/1 -> Gain/1
  Integrator/1 -> Square Root/1, h/1
  q/1 -> Sum/1
  Gain/1 -> Integrator/1
  Product/1 -> qe/1, Sum/2
  Square Root/1 -> Product/1
  C/1 -> Product/2

== system Proiect/Sistem1/Amplificator ==
  ua : Inport
  Constant : Constant  Value=8.1
  Gain : Gain  Gain=2.2
  Gain1 : Gain  Gain=2.2
  Gain2 : Gain  Gain=5
  Saturation : Saturate  UpperLimit=22  LowerLimit=0
  Sum : Sum  Inputs=|++
  Sum1 : Sum  Inputs=|+-
  Switch : Switch  Threshold=8.1  SaturateOnIntegerOverflow=off  InputSameDT=off
  um : Outport
  wires:
  Switch/1 -> Saturation/1
  ua/1 -> Switch/2, Gain/1, Sum1/1, Gain1/1
  Gain1/1 -> Sum/1
  Gain2/1 -> Sum/2
  Saturation/1 -> um/1
  Gain/1 -> Switch/3
  Constant/1 -> Sum1/2
  Sum1/1 -> Gain2/1
  Sum/1 -> Switch/1
